simulink model "SimEstanqueNN"  (R2020a)
settings: Solver=ode45  StartTime=0.0  StopTime=2000  RelTol=1e-3
values from neighbouring files (symbols this model uses):
  tescalon = 180    [ModelPredictiveControlNN.m]
settings Model: Creator=rober  LastModifiedBy=EO
settings SolverCC: ZeroCrossAlgorithm=Adaptive
settings DataIOCC: SaveFormat=StructureWithTime  ReturnWorkspaceOutputs=off
settings OptimizationCC: LifeSpan=inf
settings DebuggingCC: IgnoredZcDiagnostic=none  SFExecutionAtInitializationDiag=none  ArithmeticOperatorsInVariantConditions=warning
settings HardwareCC: ProdBitPerSizeT=32  ProdBitPerPtrDiffT=32  ProdWordSize=32  ProdHWDeviceType=Specified
settings SFSimCC: CustomCodeUndefinedFunction=UseInterfaceOnly
settings CodeAppCC: StateflowObjectComments=on

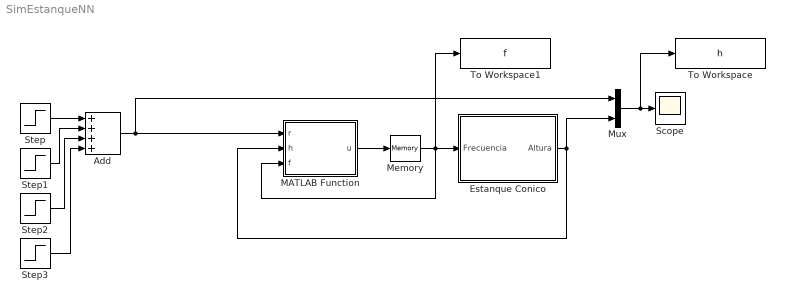
== system SimEstanqueNN ==
  Add : Sum  Inputs=++++
  Estanque Conico : Subsystem
  MATLAB Function : MATLAB Function  TreatAsAtomicUnit=on  SystemSampleTime=10
      settings: MinAlgLoopOccurrences=on
  Memory : Memory
  Mux : Mux  Inputs=2
  Scope : Scope
  Step : Step  Time=0  After=25  SampleTime=0
  Step1 : Step  Time=tescalon  After=10  SampleTime=0
  Step2 : Step  Time=2*tescalon  After=-5  SampleTime=0
  Step3 : Step  Time=4*tescalon  After=15  SampleTime=0
  To Workspace : ToWorkspace  VariableName=h  SampleTime=-1
  To Workspace1 : ToWorkspace  VariableName=f  SampleTime=-1
  wires:
  Step/1 -> Add/1
  Step1/1 -> Add/2
  Step2/1 -> Add/3
  Step3/1 -> Add/4
  Estanque Conico/1(Altura) -> Mux/2, MATLAB Function/2(h)
  Add/1 -> Mux/1, MATLAB Function/1(r)
  MATLAB Function/1(u) -> Memory/1
  Memory/1 -> To Workspace1/1, MATLAB Function/3(f), Estanque Conico/1(Frecuencia)
  Mux/1 -> To Workspace/1, Scope/1

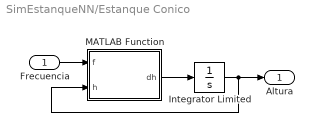
== system SimEstanqueNN/Estanque Conico ==
  Frecuencia : Inport
  Integrator Limited : Integrator  InitialCondition=20  LimitOutput=on  LowerSaturationLimit=0
  MATLAB Function : MATLAB Function  TreatAsAtomicUnit=on
  Altura : Outport
  wires:
  Integrator Limited/1 -> MATLAB Function/2(h), Altura/1
  MATLAB Function/1(dh) -> Integrator Limited/1
  Frecuencia/1 -> MATLAB Function/1(f)

== matlab function SimEstanqueNN/MATLAB Function ==
  data: r input; u output; h input; f input
function u = Controlador(r,h,f)

% coder.extrinsic('ControladorOptEuler');
coder.extrinsic('ControladorOptNN');
u=0;
% u=ControladorOptEuler(r,h,f);
u=ControladorOptNN(r,h,f);
end

== matlab function SimEstanqueNN/Estanque Conico/MATLAB Function ==
  data: f input; dh output; h input
function dh = fcn(f,h)
Fin=5.43*f+78.23;
Fout=20.21*sqrt(h);
Num=Fin-Fout;
Den=0.63*h^2+11.4*h+17.1;
dh = real(Num/Den);
